simulink model "drone_position_estimate_discrete"  (R2020b)
settings: Solver=VariableStepAuto  StartTime=0.0  StopTime=10  RelTol=1e-3
undefined symbols (not defined in the file): A, B, B_discrete, C, D, D_discrete, F_discrete, G, gps, h, H_discrete, h_plant, L, Q, R, reference, sat_max, sat_min, wind_final_value, wind_initial_value, wind_steptime, x0, x0_observer
settings Model: Creator=lucas  LastModifiedBy=lucas

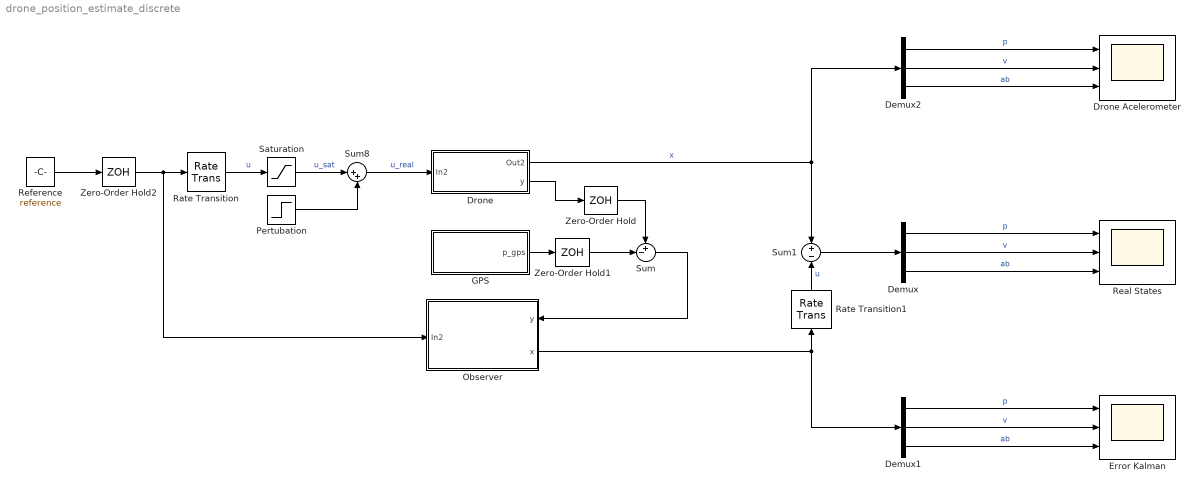
== system drone_position_estimate_discrete ==
  Demux : Demux  Outputs=3
  Demux1 : Demux  Outputs=3
  Demux2 : Demux  Outputs=3
  Drone : Subsystem
  Drone Acelerometer : Scope  NumInputPorts=3
  Error Kalman : Scope  NumInputPorts=3
  GPS : Subsystem
  Observer : Subsystem
      settings: PortSchema="{\"entries\":[{\"content\":{\"sides\":[{\"content\":{\"connectorIds\":[\"In1\"]},\"type\":\"ConnectorPlacement.EquallySpacedRectSide\",\"uuid\":\"b6dae28a-5485-44ef-84e6-2d14792229e7\"},{\"content\":{\"connectorIds\":[\"In2\",\"Out1\"],\"side\":\"RIGHT\"},\"type\":\"ConnectorPlacement.EquallySpacedRectSide\",\"uuid\":\"53a86c87-87d1-415f-9895-91b2b6ac7daf\"},{\"content\":{\"connectorIds\":[],\"side\":\"TOP\"},\"type\":\"ConnectorPlacement.EquallySpacedRectSide\",\"uuid\":\"c2916f3e-51bf-40f4-b6cd-eee6b60c38ec\"},{\"content\":{\"connectorIds\":[],\"side\":\"HIDDEN\"},\"type\":\"ConnectorPlacement.EquallySpacedRectSide\",\"uuid\":\"c85aafdf-e330-4d8d-a14a-206e12d7d836\"}]},\"type\":\"ConnectorPlacement.EquallySpacedConnector\",\"uuid\":\"08a8a426-31b9-42c2-8372-de3a4deaf2af\"}],\"packageUris\":[\"http://schema.mathworks.com/mf0/Connector/R2020b\"],\"version\":\"1.0\"}"
  Pertubation : Step  Time=wind_steptime  Before=wind_initial_value  After=wind_final_value  SampleTime=h_plant
  Rate Transition : RateTransition  Integrity=off  OutPortSampleTimeMultiple=0.01  OutPortSampleTime=h_plant
  Rate Transition1 : RateTransition  Integrity=off  OutPortSampleTimeMultiple=0.01
  Real States : Scope  NumInputPorts=3
  Reference : Constant  Value=reference  SampleTime=h
  Saturation : Saturate  UpperLimit=sat_max  LowerLimit=sat_min
  Sum : Sum  Inputs=+-|
  Sum1 : Sum  Inputs=+|-
  Sum8 : Sum  Inputs=|++
  Zero-Order Hold : ZeroOrderHold  SampleTime=h
  Zero-Order Hold1 : ZeroOrderHold  SampleTime=h
  Zero-Order Hold2 : ZeroOrderHold  SampleTime=h
  wires:
  Reference/1 -> Zero-Order Hold2/1
  Demux1/2 -> Error Kalman/2  "v"
  Demux2/2 -> Drone Acelerometer/2  "v"
  Demux2/1 -> Drone Acelerometer/1  "p"
  Saturation/1 -> Sum8/1  "u_sat"
  Rate Transition/1 -> Saturation/1  "u"
  Sum8/1 -> Drone/1(In2)  "u_real"
  Demux1/1 -> Error Kalman/1  "p"
  Demux1/3 -> Error Kalman/3  "ab"
  Demux2/3 -> Drone Acelerometer/3  "ab"
  Sum/1 -> Observer/2(y)
  Demux/1 -> Real States/1  "p"
  Sum1/1 -> Demux/1
  Pertubation/1 -> Sum8/2
  Demux/2 -> Real States/2  "v"
  Drone/1(Out2) -> Demux2/1, Sum1/1  "x"
  Demux/3 -> Real States/3  "ab"
  Observer/1(x) -> Rate Transition1/1, Demux1/1
  Drone/2(y) -> Zero-Order Hold/1
  Zero-Order Hold/1 -> Sum/1
  Zero-Order Hold1/1 -> Sum/2
  GPS/1(p_gps) -> Zero-Order Hold1/1
  Zero-Order Hold2/1 -> Observer/1(In2), Rate Transition/1
  Rate Transition1/1 -> Sum1/2  "u"

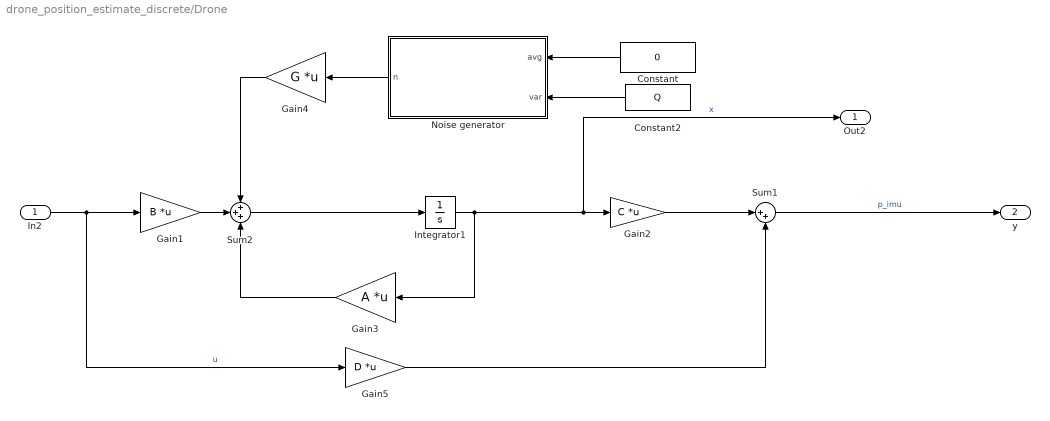
== system drone_position_estimate_discrete/Drone ==
  In2 : Inport
  Constant : Constant  Value=0  VectorParams1D=off
  Constant2 : Constant  Value=Q
  Gain1 : Gain  Gain=B  Multiplication=Matrix(K*u) (u vector)
  Gain2 : Gain  Gain=C  Multiplication=Matrix(K*u) (u vector)
  Gain3 : Gain  Gain=A  Multiplication=Matrix(K*u) (u vector)
  Gain4 : Gain  Gain=G  Multiplication=Matrix(K*u) (u vector)
  Gain5 : Gain  Gain=D  Multiplication=Matrix(K*u) (u vector)
  Integrator1 : Integrator  InitialCondition=x0
  Noise generator : MATLAB Function  TreatAsAtomicUnit=on
  Sum1 : Sum  Inputs=|++
  Sum2 : Sum  Inputs=+++
  Out2 : Outport
  y : Outport  Port=2
  wires:
  Sum2/1 -> Integrator1/1
  Gain2/1 -> Sum1/1
  Sum1/1 -> y/1  "p_imu"
  In2/1 -> Gain5/1, Gain1/1  "u"
  Integrator1/1 -> Gain3/1, Out2/1, Gain2/1  "x"
  Gain1/1 -> Sum2/2
  Gain3/1 -> Sum2/3
  Noise generator/1(n) -> Gain4/1
  Gain4/1 -> Sum2/1
  Constant/1 -> Noise generator/1(avg)
  Constant2/1 -> Noise generator/2(var)
  Gain5/1 -> Sum1/2

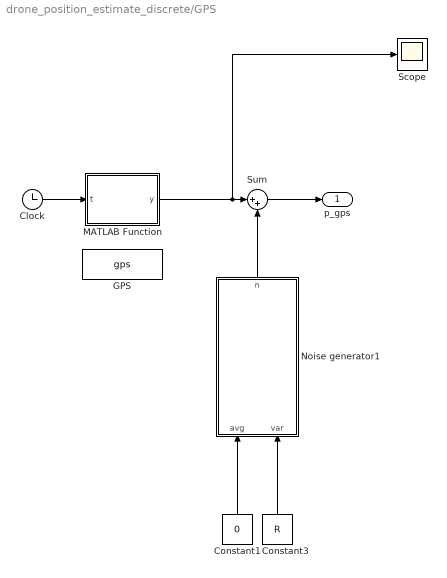
== system drone_position_estimate_discrete/GPS ==
  Clock : Clock
  Constant1 : Constant  Value=0
  Constant3 : Constant  Value=R
  GPS : Constant  Value=gps  VectorParams1D=off  SampleTime=h
  MATLAB Function : MATLAB Function  TreatAsAtomicUnit=on
  Noise generator1 : MATLAB Function  TreatAsAtomicUnit=on
  Scope : Scope
  Sum : Sum  Inputs=|++
  p_gps : Outport
  wires:
  Noise generator1/1(n) -> Sum/2
  Constant3/1 -> Noise generator1/2(var)
  Constant1/1 -> Noise generator1/1(avg)
  Sum/1 -> p_gps/1
  Clock/1 -> MATLAB Function/1(t)
  MATLAB Function/1(y) -> Scope/1, Sum/1

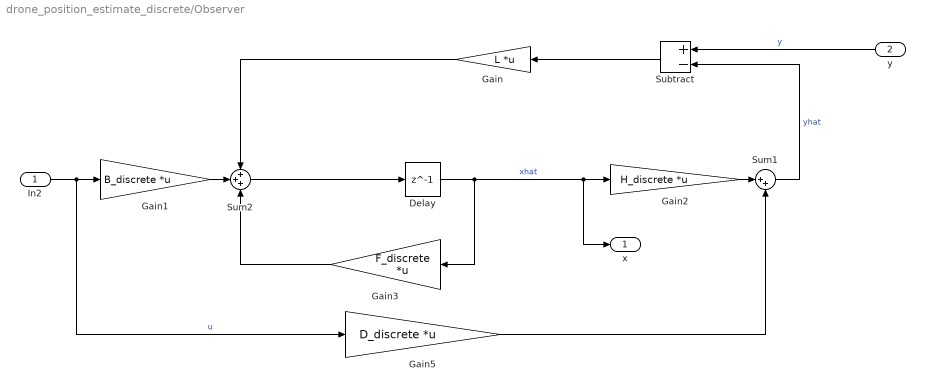
== system drone_position_estimate_discrete/Observer ==
  In2 : Inport
  y : Inport  Port=2
  Delay : Delay  DelayLength=1  InitialCondition=x0_observer
  Gain : Gain  Gain=L  Multiplication=Matrix(K*u) (u vector)
  Gain1 : Gain  Gain=B_discrete  Multiplication=Matrix(K*u) (u vector)
  Gain2 : Gain  Gain=H_discrete  Multiplication=Matrix(K*u) (u vector)
  Gain3 : Gain  Gain=F_discrete  Multiplication=Matrix(K*u) (u vector)
  Gain5 : Gain  Gain=D_discrete  Multiplication=Matrix(K*u) (u vector)
  Subtract : Sum  Inputs=+-
  Sum1 : Sum  Inputs=|++
  Sum2 : Sum  Inputs=+++
  x : Outport
  wires:
  Gain5/1 -> Sum1/2
  In2/1 -> Gain5/1, Gain1/1  "u"
  Sum2/1 -> Delay/1
  Gain3/1 -> Sum2/3
  Delay/1 -> Gain3/1, x/1, Gain2/1  "xhat"
  Gain1/1 -> Sum2/2
  Gain2/1 -> Sum1/1
  y/1 -> Subtract/1  "y"
  Sum1/1 -> Subtract/2  "yhat"
  Subtract/1 -> Gain/1
  Gain/1 -> Sum2/1

== matlab function drone_position_estimate_discrete/GPS/Noise generator1 ==
  data: avg input; n output; var input
function n = generate_gaussian_noise(avg, var)
n = avg + var*randn(length(var), 1);

== matlab function drone_position_estimate_discrete/Drone/Noise generator ==
  data: avg input; n output; var input
function n = generate_gaussian_noise(avg, var)
n = avg + var*randn(length(var), 1);

== matlab function drone_position_estimate_discrete/GPS/MATLAB Function ==
  data: t input; y output; x0 parameter
function y = fcn(t, x0)
    y = [0;0;(x0(3) + x0(6)*t -9.98*(t^2)/2)];
